simulink model "exampe_1_r2016a"  (R2016a)
settings: Solver=FixedStepAuto  SolverMode=SingleTasking  StartTime=0.0  StopTime=inf  RelTol=1e-3
libraries: aerolibanimutils x1
settings Model: Creator=Desktop-dds  LastModifiedBy=Desktop-dds
settings DebuggingCC: SFUnexpectedBacktrackingDiag=error  SFNoUnconditionalDefaultTransitionDiag=error
settings SFSimCC: SimUseLocalCustomCode=on
settings RTWCC: RTWUseLocalCustomCode=on
settings GRTTargetCC: TargetLangStandard=C99 (ISO)  GeneratePreprocessorConditionals=Use local settings
settings ConfigComp: CovMetricSettings=dwe  CovHtmlReporting=off  CovSaveCumulativeToWorkspaceVar=off  CovSaveSingleToWorkspaceVar=off  CovExternalEMLEnable=on

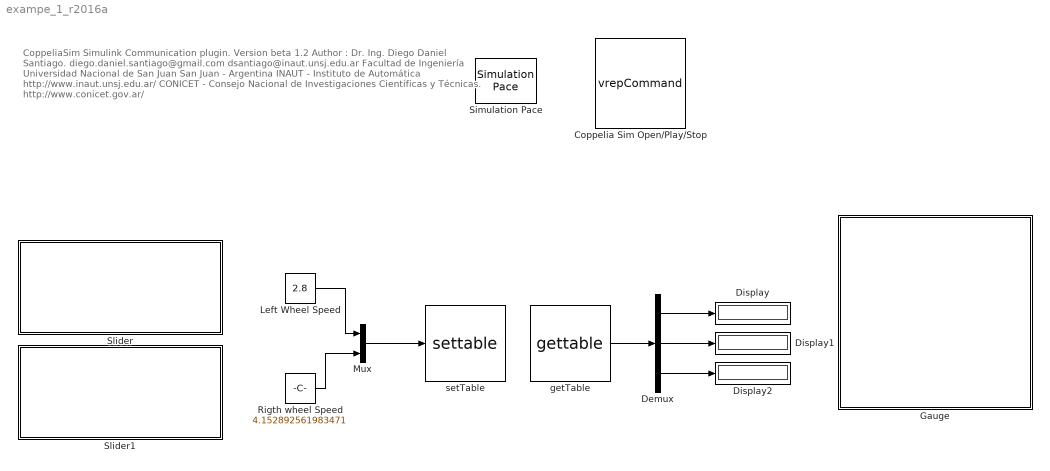
== system exampe_1_r2016a ==
  note: CoppeliaSim Simulink Communication plugin.
      | Version beta 1.2
      | Author : Dr. Ing. Diego Daniel Santiago.
      | diego.daniel.santiago@gmail.com
      | dsantiago@inaut.unsj.edu.ar
      | Facultad de Ingeniería
      | Universidad Nacional de San Juan
      | San Juan - Argentina
      |
      | INAUT - Instituto de Automática
      | http://www.inaut.unsj.edu.ar/
      | CONICET - Consejo Nacional de Investigaciones Científicas y Técnicas.
      | http://www.conicet.gov.ar/
  Coppelia Sim Open/Play/Stop : S-Function  FunctionName=vrepCommand  Parameters=scene  SFunctionDeploymentMode=off  EnableBusSupport=off  mask{scene='example1.ttt'}
      mask prompts: scene "V-rep Scene Name"
      mask Display: image('play_stop.png')
  Demux : Demux  Outputs=3
  Display : Display
  Display1 : Display
  Display2 : Display
  Gauge : Subsystem  DialogController=hmiCreateDDGDialog  IsWebBlock=on  mask(MWDashboardBlock){webBlockId=0ee06b22-4159-4906-bd28-e31a6fc0223c, webBlockType=circulargauge, ShowInLibBrowser=on, ShowInitialText=on, HMISrcModelName=example1_16a}
      mask prompts: webBlockId "WebBlock Id"; webBlockType "WebBlock Type"; HMISrcModelName "Source Model"
      mask help: Display an input value on a circular scale.
      mask Help: helpview([docroot '/mapfiles/simulink.map'], 'hmi_gauge')
      mask Display:
      | if strcmp(get_param(bdroot(gcb),'BlockDiagramType'),'library')
      |  image([(matlabroot) '/toolbox/simulink/hmi/icons/CircularGauge.png'])
      | end
  Left Wheel Speed : Constant  Value=2.8
  Mux : Mux  Inputs=2
  Rigth wheel Speed : Constant  Value=4.152892561983471
  Simulation Pace : aerolibanimutils/Simulation Pace  SimulationPace=1  SleepMode=Auto  OutputPaceError=off  SampleTime=1/30
  Slider : Subsystem  DialogController=hmiCreateDDGDialog  IsWebBlock=on  mask(MWDashboardBlock){webBlockId=2551fdc4-2f0b-4f19-a239-5c2f2d6547ce, webBlockType=slider, ShowInLibBrowser=on, ShowInitialText=on, HMISrcModelName=example1_16a}
      mask prompts: webBlockId "WebBlock Id"; webBlockType "WebBlock Type"; HMISrcModelName "Source Model"
      mask help: Set value to tune parameters or variables.
      mask Help: helpview([docroot '/mapfiles/simulink.map'], 'hmi_slider')
      mask Display:
      | if strcmp(get_param(bdroot(gcb),'BlockDiagramType'),'library')
      |  image([(matlabroot) '/toolbox/simulink/hmi/icons/Slider.png'])
      | end
  Slider1 : Subsystem  DialogController=hmiCreateDDGDialog  IsWebBlock=on  mask(MWDashboardBlock){webBlockId=1051b2d4-36ba-40a2-a2a5-2fe0f34f4968, webBlockType=slider, ShowInLibBrowser=on, ShowInitialText=on, HMISrcModelName=example1_16a}
      mask prompts: webBlockId "WebBlock Id"; webBlockType "WebBlock Type"; HMISrcModelName "Source Model"
      mask help: Set value to tune parameters or variables.
      mask Help: helpview([docroot '/mapfiles/simulink.map'], 'hmi_slider')
      mask Display:
      | if strcmp(get_param(bdroot(gcb),'BlockDiagramType'),'library')
      |  image([(matlabroot) '/toolbox/simulink/hmi/icons/Slider.png'])
      | end
  getTable : S-Function  FunctionName=gettable  Parameters=tname  SFunctionDeploymentMode=off  EnableBusSupport=off  mask{tname='sens'}
      mask prompts: tname "Table Name"
      mask DialogControl DescGroupVar Prompt: GetData
      mask DialogControl DescTextVar Prompt: Gets the data from a table declared in CoppeliaSim
      mask Display: image("CoppeliaSim.png")
  setTable : S-Function  FunctionName=settable  Parameters=tname  SFunctionDeploymentMode=off  EnableBusSupport=off  mask{tname='act'}
      mask prompts: tname "Table Name"
      mask DialogControl DescGroupVar Prompt: SetData
      mask DialogControl DescTextVar Prompt: Copy the input data into a table declared in CoppeliaSim
      mask Display: image("CoppeliaSim.png")
  wires:
  Mux/1 -> setTable/1
  Left Wheel Speed/1 -> Mux/1
  Rigth wheel Speed/1 -> Mux/2
  getTable/1 -> Demux/1
  Demux/1 -> Display/1
  Demux/2 -> Display1/1
  Demux/3 -> Display2/1

== system exampe_1_r2016a/Gauge ==

== system exampe_1_r2016a/Slider ==

== system exampe_1_r2016a/Slider1 ==
